simulink model "BGF"  (R2022b)
settings: Solver=FixedStepAuto  StartTime=0.0  StopTime=1000000  FixedStep=0.1  RelTol=1e-3
values from neighbouring files (symbols this model uses):
  A = [1 10 35 50 24]    [parameter.m]
  A_0 = [1 11 36 51 25]    [parameter.m]
  A_F = [1 1 1 1]    [parameter.m]
  B = [10]    [parameter.m]
libraries: matrix_library x2
settings Model: Creator=iran sistem  LastModifiedBy=110

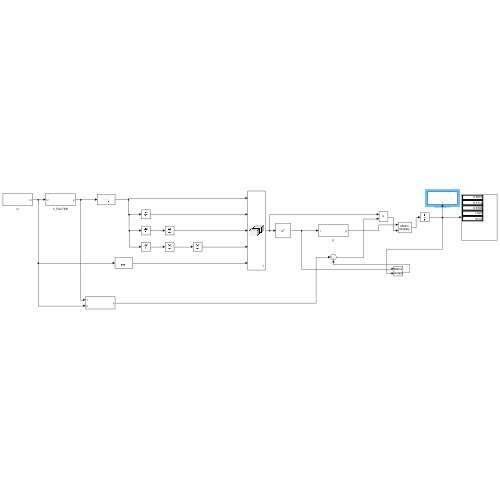
[thumbnail: Simulink's stored preview of the top-level diagram]
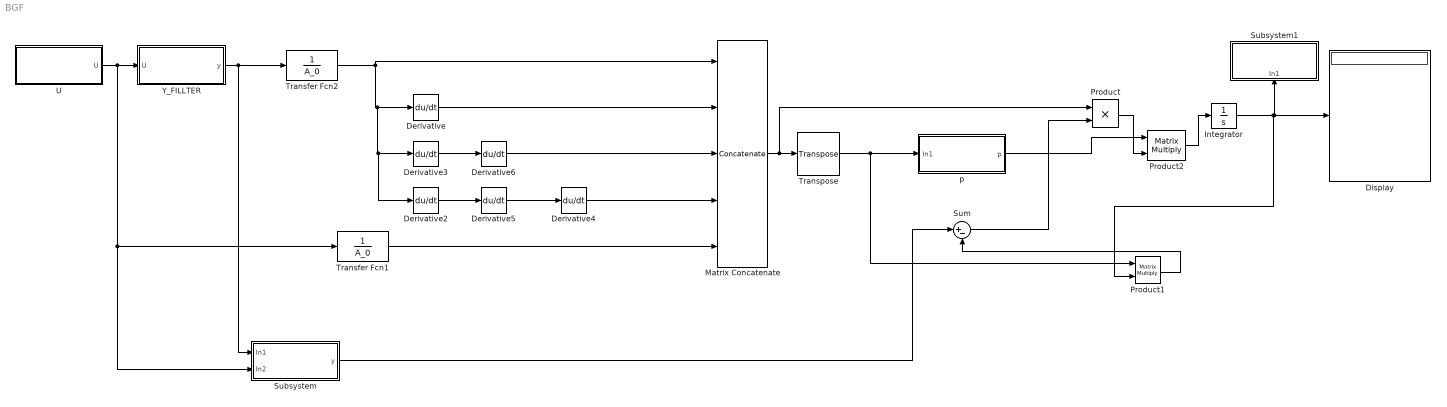
== system BGF ==
  Derivative{,2..6} (6 alike) : Derivative
  Display : Display
  Integrator : Integrator
  Matrix Concatenate : Concatenate  NumInputs=5  Mode=Multidimensional array
  Product : Product
  Product1 : Product  Multiplication=Matrix(*)
  Product2 : Product  Multiplication=Matrix(*)
  Subsystem : Subsystem
  Subsystem1 : Subsystem
      settings: PortSchema="{\"entries\":[{\"content\":{\"sides\":[{\"content\":{\"connectorIds\":[]},\"type\":\"ConnectorPlacement.EquallySpacedRectSide\",\"uuid\":\"52b6fdf9-1802-49ef-85fd-54fc755b953c\"},{\"content\":{\"connectorIds\":[],\"side\":\"RIGHT\"},\"type\":\"ConnectorPlacement.EquallySpacedRectSide\",\"uuid\":\"96d61da8-85e0-4c2c-a1b4-af071e987e17\"},{\"content\":{\"connectorIds\":[],\"side\":\"TOP\"},\"type\":\"ConnectorPlacement.EquallySpacedRectSide\",\"uuid\":\"56674c31-5d8f-4ec5-8559-e3ea3a9ef119\"},{\"content\":{\"connectorIds\":[\"In1\"],\"side\":\"BOTTOM\"},\"type\":\"ConnectorPlacement.EquallySpacedRectSide\",\"uuid\":\"5dd4f15e-9996-46af-9591-1fc4d24af015\"}]},\"type\":\"ConnectorPlacement.EquallySpacedConnector\",\"uuid\":\"764673e8-5feb-4a89-8854-6cef5b8dd69e\"}],\"packageUris\":[\"http://schema.mathworks.com/mf0/Connector/R2020b\"],\"version\":\"1.0\"}"
  Sum : Sum  Inputs=|+-
  Transfer Fcn1 : TransferFcn  Denominator=A_0
  Transfer Fcn2 : TransferFcn  Denominator=A_0
  Transpose : matrix_library/Transpose
  U : Subsystem
  Y_FILLTER : Subsystem
  p : Subsystem
  wires:
  p/1(p) -> Product2/1
  Product2/1 -> Integrator/1
  Derivative2/1 -> Derivative5/1
  Transfer Fcn1/1 -> Matrix Concatenate/5
  Derivative/1 -> Matrix Concatenate/2
  Derivative5/1 -> Derivative4/1
  Product1/1 -> Sum/2
  Transfer Fcn2/1 -> Derivative2/1, Derivative3/1, Derivative/1, Matrix Concatenate/1
  Product/1 -> Product2/2
  Transpose/1 -> Product1/1, p/1(In1)
  Derivative3/1 -> Derivative6/1
  Matrix Concatenate/1 -> Product/1, Transpose/1
  Y_FILLTER/1(y) -> Subsystem/1(In1), Transfer Fcn2/1
  Derivative6/1 -> Matrix Concatenate/3
  Integrator/1 -> Subsystem1/1(In1), Display/1, Product1/2
  Derivative4/1 -> Matrix Concatenate/4
  U/1(U) -> Subsystem/2(In2), Transfer Fcn1/1, Y_FILLTER/1(U)
  Sum/1 -> Product/2
  Subsystem/1(y) -> Sum/1

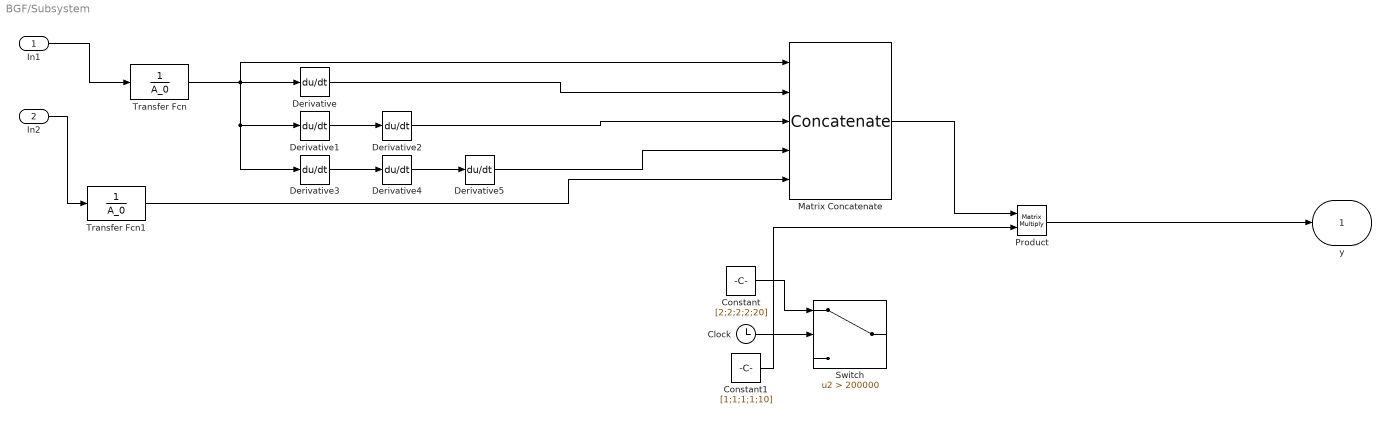
== system BGF/Subsystem ==
  In1 : Inport
  In2 : Inport  Port=2
  Clock : Clock
  Constant : Constant  Value=[2;2;2;2;20]
  Constant1 : Constant  Value=[1;1;1;1;10]
  Derivative{,1..5} (6 alike) : Derivative
  Matrix Concatenate : Concatenate  NumInputs=5  Mode=Multidimensional array  ConcatenateDimension=2
  Product : Product  Multiplication=Matrix(*)
  Switch : Switch  Criteria=u2 > Threshold  Threshold=200000  SaturateOnIntegerOverflow=off  InputSameDT=off
  Transfer Fcn : TransferFcn  Denominator=A_0
  Transfer Fcn1 : TransferFcn  Denominator=A_0
  y : Outport
  wires:
  Product/1 -> y/1
  Matrix Concatenate/1 -> Product/1
  In1/1 -> Transfer Fcn/1
  In2/1 -> Transfer Fcn1/1
  Transfer Fcn/1 -> Derivative3/1, Derivative1/1, Matrix Concatenate/1, Derivative/1
  Derivative/1 -> Matrix Concatenate/2
  Derivative1/1 -> Derivative2/1
  Derivative2/1 -> Matrix Concatenate/3
  Derivative3/1 -> Derivative4/1
  Derivative4/1 -> Derivative5/1
  Derivative5/1 -> Matrix Concatenate/4
  Transfer Fcn1/1 -> Matrix Concatenate/5
  Clock/1 -> Switch/2
  Constant/1 -> Switch/1
  Constant1/1 -> Product/2

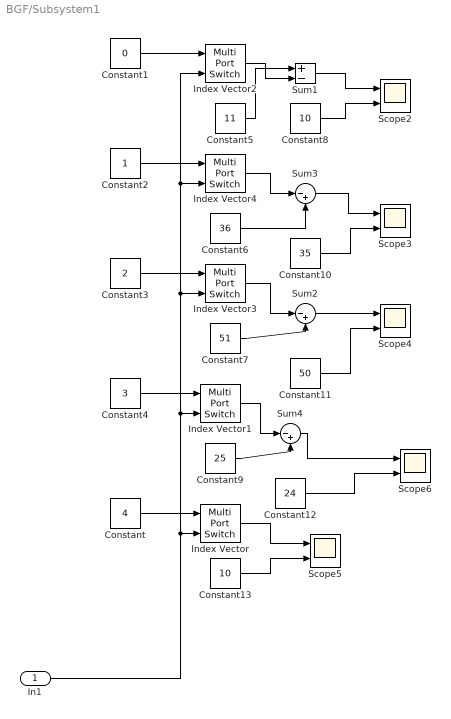
== system BGF/Subsystem1 ==
  In1 : Inport
  Constant : Constant  Value=4
  Constant1 : Constant  Value=0
  Constant10 : Constant  Value=35
  Constant11 : Constant  Value=50
  Constant12 : Constant  Value=24
  Constant13 : Constant  Value=10
  Constant2 : Constant
  Constant3 : Constant  Value=2
  Constant4 : Constant  Value=3
  Constant5 : Constant  Value=11
  Constant6 : Constant  Value=36
  Constant7 : Constant  Value=51
  Constant8 : Constant  Value=10
  Constant9 : Constant  Value=25
  Index Vector{,1..4} (5 alike) : MultiPortSwitch  DataPortOrder=Zero-based contiguous  Inputs=1  zeroidx=on  SaturateOnIntegerOverflow=off  InputSameDT=off
  Scope{2..6} (5 alike) : Scope  NumInputPorts=2
  Sum1 : Sum  Inputs=|+-
  Sum2 : Sum  Inputs=|-+
  Sum3 : Sum  Inputs=|-+
  Sum4 : Sum  Inputs=|-+
  wires:
  Constant1/1 -> Index Vector2/1
  In1/1 -> Index Vector3/2, Index Vector2/2, Index Vector4/2, Index Vector1/2, Index Vector/2
  Constant3/1 -> Index Vector3/1
  Constant/1 -> Index Vector/1
  Constant2/1 -> Index Vector4/1
  Constant11/1 -> Scope4/2
  Constant9/1 -> Sum4/2
  Constant4/1 -> Index Vector1/1
  Index Vector1/1 -> Sum4/1
  Constant8/1 -> Scope2/2
  Constant7/1 -> Sum2/2
  Constant12/1 -> Scope6/2
  Sum3/1 -> Scope3/1
  Index Vector2/1 -> Sum1/2
  Sum2/1 -> Scope4/1
  Index Vector/1 -> Scope5/1
  Sum4/1 -> Scope6/1
  Constant5/1 -> Sum1/1
  Index Vector4/1 -> Sum3/1
  Constant10/1 -> Scope3/2
  Index Vector3/1 -> Sum2/1
  Sum1/1 -> Scope2/1
  Constant13/1 -> Scope5/2
  Constant6/1 -> Sum3/2

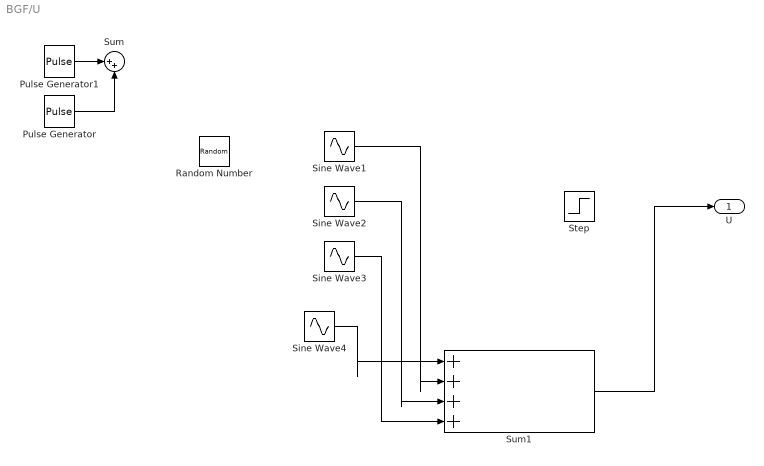
== system BGF/U ==
  Pulse Generator : DiscretePulseGenerator  PulseType=Time based  Amplitude=-1  Period=20  PulseWidth=50
  Pulse Generator1 : DiscretePulseGenerator  PulseType=Time based  Period=20  PulseWidth=50
  Random Number : RandomNumber  SampleTime=0.1
  Sine Wave1 : Sin  Frequency=5  SampleTime=0
  Sine Wave2 : Sin  Frequency=2  SampleTime=0
  Sine Wave3 : Sin  Frequency=3  SampleTime=0
  Sine Wave4 : Sin  SampleTime=0
  Step : Step  SampleTime=0
  Sum : Sum  Inputs=|++
  Sum1 : Sum  Inputs=|++++
  U : Outport
  wires:
  Pulse Generator1/1 -> Sum/1
  Pulse Generator/1 -> Sum/2
  Sine Wave1/1 -> Sum1/2
  Sine Wave2/1 -> Sum1/3
  Sine Wave3/1 -> Sum1/4
  Sine Wave4/1 -> Sum1/1
  Sum1/1 -> U/1

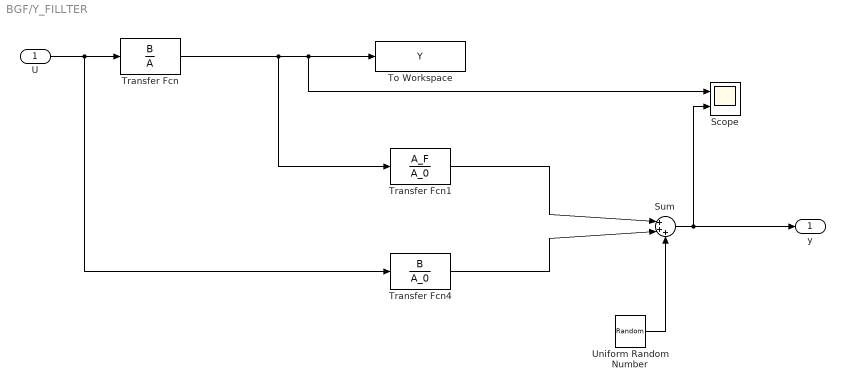
== system BGF/Y_FILLTER ==
  U : Inport
  Scope : Scope  NumInputPorts=2
  Sum : Sum  Inputs=|+++
  To Workspace : ToWorkspace  VariableName=Y  SaveFormat=Timeseries  SampleTime=-1
  Transfer Fcn : TransferFcn  Numerator=B  Denominator=A
  Transfer Fcn1 : TransferFcn  Numerator=A_F  Denominator=A_0
  Transfer Fcn4 : TransferFcn  Numerator=B  Denominator=A_0
  Uniform Random Number : UniformRandomNumber  SampleTime=0.1
  y : Outport
  wires:
  U/1 -> Transfer Fcn4/1, Transfer Fcn/1
  Transfer Fcn/1 -> Transfer Fcn1/1, Scope/1, To Workspace/1
  Transfer Fcn1/1 -> Sum/1
  Transfer Fcn4/1 -> Sum/2
  Sum/1 -> y/1, Scope/2
  Uniform Random Number/1 -> Sum/3

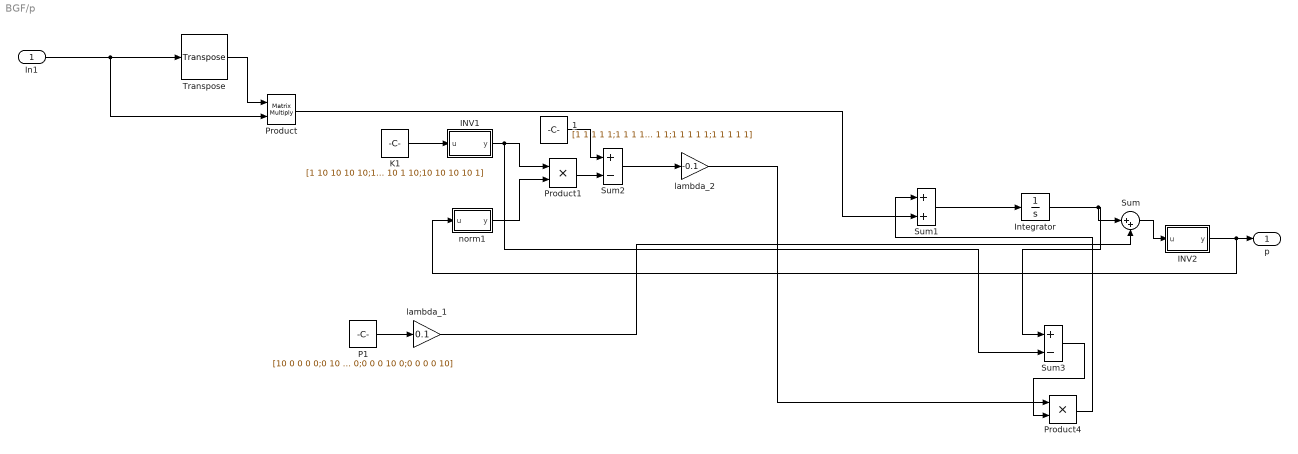
== system BGF/p ==
  In1 : Inport
  1 : Constant  Value=[1 1 1 1 1;1 1 1 1 1;1 1 1 1 1;1 1 1 1 1;1 1 1 1 1]
  INV1 : MATLAB Function  TreatAsAtomicUnit=on
  INV2 : MATLAB Function  TreatAsAtomicUnit=on
  Integrator : Integrator
  K1 : Constant  Value=[1 10 10 10 10;10 1 10 10 10;10 10 1 10 10;10 10 10 1 10;10 10 10 10 1]
  P1 : Constant  Value=[10 0 0 0 0;0 10 0 0 0;0 0 10 0 0;0 0 0 10 0;0 0 0 0 10]
  Product : Product  Multiplication=Matrix(*)
  Product1 : Product
  Product4 : Product
  Sum : Sum  Inputs=|++
  Sum1 : Sum
  Sum2 : Sum  Inputs=+-
  Sum3 : Sum  Inputs=+-
  Transpose : matrix_library/Transpose
  lambda_1 : Gain  Gain=0.1
  lambda_2 : Gain  Gain=-0.1
  norm1 : MATLAB Function  TreatAsAtomicUnit=on
  p : Outport
  wires:
  In1/1 -> Product/2, Transpose/1
  Transpose/1 -> Product/1
  P1/1 -> lambda_1/1
  INV2/1(y) -> norm1/1(u), p/1
  Product/1 -> Sum1/2
  Sum1/1 -> Integrator/1
  K1/1 -> INV1/1(u)
  INV1/1(y) -> Sum3/2, Product1/1
  norm1/1(y) -> Product1/2
  Product1/1 -> Sum2/2
  1/1 -> Sum2/1
  Sum2/1 -> lambda_2/1
  Integrator/1 -> Sum/1, Sum3/1
  Sum3/1 -> Product4/2
  Product4/1 -> Sum1/1
  lambda_1/1 -> Sum/2
  Sum/1 -> INV2/1(u)
  lambda_2/1 -> Product4/1

== matlab function BGF/p/INV2 ==
  data: u input; y output
function y = fcn(u)

y = inv(u);

== matlab function BGF/p/norm1 ==
  data: u input; y output
function y = fcn(u)

y = norm(u);

== matlab function BGF/p/INV1 ==
  data: u input; y output
function y = fcn(u)

y = inv(u);
